simulink model "lift_model_5_floor"  (R2020b)
settings: Solver=VariableStepAuto  StartTime=0.0  StopTime=30  RelTol=1e-3
settings Model: Creator=153  LastModifiedBy=153

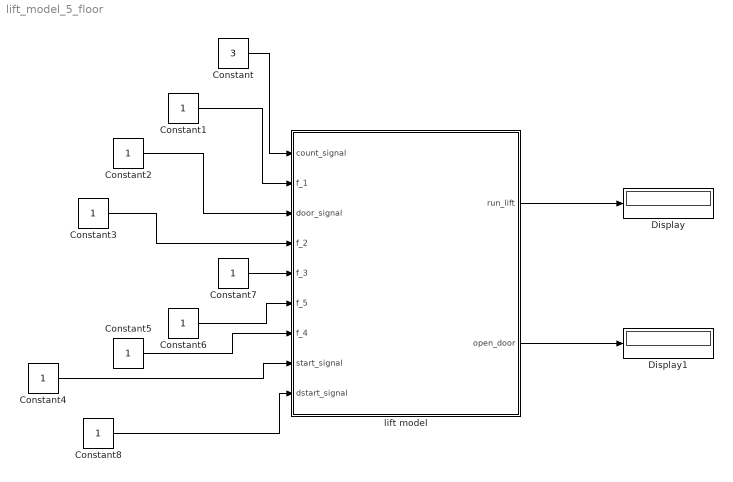
== system lift_model_5_floor ==
  Constant : Constant  Value=3
  Constant{1..8} (8 alike) : Constant
  Display : Display
  Display1 : Display
  lift model : Stateflow chart  TreatAsAtomicUnit=on
  wires:
  lift model/1(run_lift) -> Display/1
  lift model/2(open_door) -> Display1/1
  Constant/1 -> lift model/1(count_signal)
  Constant1/1 -> lift model/2(f_1)
  Constant2/1 -> lift model/3(door_signal)
  Constant3/1 -> lift model/4(f_2)
  Constant4/1 -> lift model/8(start_signal)
  Constant5/1 -> lift model/7(f_4)
  Constant6/1 -> lift model/6(f_5)
  Constant7/1 -> lift model/5(f_3)
  Constant8/1 -> lift model/9(dstart_signal)

== stateflow chart lift_model_5_floor/lift model ==
  state lift_operation [parallel]
    settings: executionOrder=1
    state idle
      en: open_door=0;
    state standmode
    state fifth
      en:run_lift=0;
      open_door=1;
      on after(5,sec):
      open_door=0;
    state enterlift_first
      en:run_lift=0;
      on after(3,sec):
      open_door=0;
    state stop
      on after(10,sec): open_door=0;
    state third
      en:run_lift=0;open_door=1;
      on after(5,sec):
      open_door=0;
    state second
      en: run_lift=0;
      open_door=1;
      on after(5,sec):
      open_door=0;
    state fourth
      en:run_lift=0;
      open_door=1;
      on after(5,sec): open_door=0;
    (default) -> standmode
    (junction 9) -> idle [order 2] : [door_signal==0]
    fifth -> fifth [order 2] : [dstart_signal==0]
    idle -> enterlift_first : [door_signal==1]
    standmode -> (junction 9)
    fourth -> fifth [order 1] : [(f_5==1)]{run_lift=1;}
    fifth -> fourth [order 1] : [(dstart_signal==1)&&((f_1==1)||(f_3==1)||(f_4==1)||(f_2==1))]{run_lift=1;}
    (junction 9) -> enterlift_first [order 1] : [door_signal==1]
    enterlift_first -> stop [order 2] : [(start_signal==0)||(count_signal>5)]
    stop -> enterlift_first : [(start_signal==1)&&(in(checker.check))]
    enterlift_first -> second [order 1] : [(f_2==1)||(f_3==1)||(f_4==1)||(f_5==1)]{run_lift==1;}
    second -> enterlift_first [order 2] : [f_1==1]{run_lift=1;}
    third -> fourth [order 1] : [(f_4==1)||(f_5==1)]{run_lift=1;}
    second -> third [order 1] : [(f_3==1)||(f_4==1)||(f_5==1)]{run_lift=1;}
    third -> second [order 2] : [(f_2==1)||(f_3==1)]{run_lift=1;}
    fourth -> third [order 2] : [(f_3==1)||(f_2==1)||(f_1==1)]{run_lift==1;}
  state checker [parallel]
    settings: executionOrder=2
    state check
    state alarm
    (default) -> check
    alarm -> check : [in(lift_operation.stop)]
    check -> alarm : [in(lift_operation.enterlift_first)]
  data: count_signal input; f_1 input; door_signal input; f_2 input; f_3 input; f_5 input; f_4 input; start_signal input; run_lift output; open_door output; dstart_signal input
